simulink model "st_re_fig1"  (R2017b)
settings: Solver=VariableStepAuto  StartTime=0.0  StopTime=1  MaxStep=1e-4  RelTol=1e-3
settings Model: Creator=Administrator  LastModifiedBy=Administrator

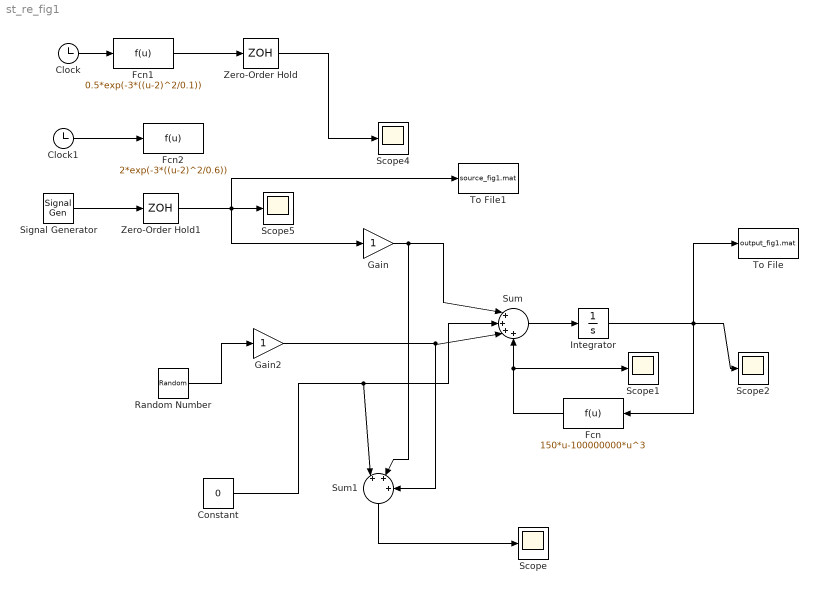
== system st_re_fig1 ==
  Clock : Clock
  Clock1 : Clock
  Constant : Constant  Value=0
  Fcn : Fcn  Expr=150*u-100000000*u^3
  Fcn1 : Fcn  Expr=0.5*exp(-3*((u-2)^2/0.1))
  Fcn2 : Fcn  Expr=2*exp(-3*((u-2)^2/0.6))
  Gain : Gain
  Gain2 : Gain
  Integrator : Integrator
  Random Number : RandomNumber  SampleTime=0.00001
  Scope{,1..2,4..5} (5 alike) : Scope
  Signal Generator : SignalGenerator  Amplitude=0.2  Frequency=15
  Sum : Sum  Inputs=|++++
  Sum1 : Sum  Inputs=|+++
  To File : ToFile  Filename=output_fig1.mat  MatrixName=output_f1  SaveFormat=Timeseries
  To File1 : ToFile  Filename=source_fig1.mat  MatrixName=source_f1  SaveFormat=Timeseries
  Zero-Order Hold : ZeroOrderHold  SampleTime=0.0001
  Zero-Order Hold1 : ZeroOrderHold  SampleTime=0.00001
  wires:
  Constant/1 -> Sum1/1, Sum/2
  Gain/1 -> Sum1/2, Sum/1
  Fcn/1 -> Sum/4, Scope1/1
  Sum/1 -> Integrator/1
  Integrator/1 -> To File/1, Scope2/1, Fcn/1
  Sum1/1 -> Scope/1
  Clock/1 -> Fcn1/1
  Clock1/1 -> Fcn2/1
  Gain2/1 -> Sum1/3, Sum/3
  Fcn1/1 -> Zero-Order Hold/1
  Zero-Order Hold/1 -> Scope4/1
  Signal Generator/1 -> Zero-Order Hold1/1
  Zero-Order Hold1/1 -> To File1/1, Gain/1, Scope5/1
  Random Number/1 -> Gain2/1
